simulink model "six_plus_six_AcmsteeringV09_main_1lf"  (R2014a)
settings: Solver=FixedStepDiscrete  StartTime=0.0  StopTime=10.0  FixedStep=0.0005  RelTol=1e-3
InitFcn:
  | Veh_Par_wxt
undefined symbols (not defined in the file or in its folder): acc_spdctl, ag_thr, B, bra_em, bra_pre_gz2, bra_pre_gz34, bra_pre_yd, brakepre_dem_data, brakeTrq_dem_data, bratrq_max, ecucoder_acal, eff_tran, ESP_switch, G, guzhang_lf, guzhang_lm, guzhang_lr, guzhang_rf, guzhang_rm, guzhang_rr, kd1, kd2, ki1, ki2, kp1, kp2, L, myFIS, premax, Radius, RC_switch, s_opt_yi, s_opt_zhuan, s_opt_zhuan_add, s_opt_zhuan_table, spd_map_mot, spd_spdctl, speed_thr_park, TCS_switch, tras_ratio, trq_map_mot, trqmax_yd, trqmax_zx, trqmaxneg, v_gain, v_table, v_thr_park, zhidong_bianmazhi, zhidong_down, zhidong_up, zhidong_youmen, zhuanxiang_bianmazhi, zhuanxiang_down, zhuanxiang_up, zhuanxiang_youmen
libraries: simulink x980, ec5744lib x59, fuzblock x2
(part 22 of 25)

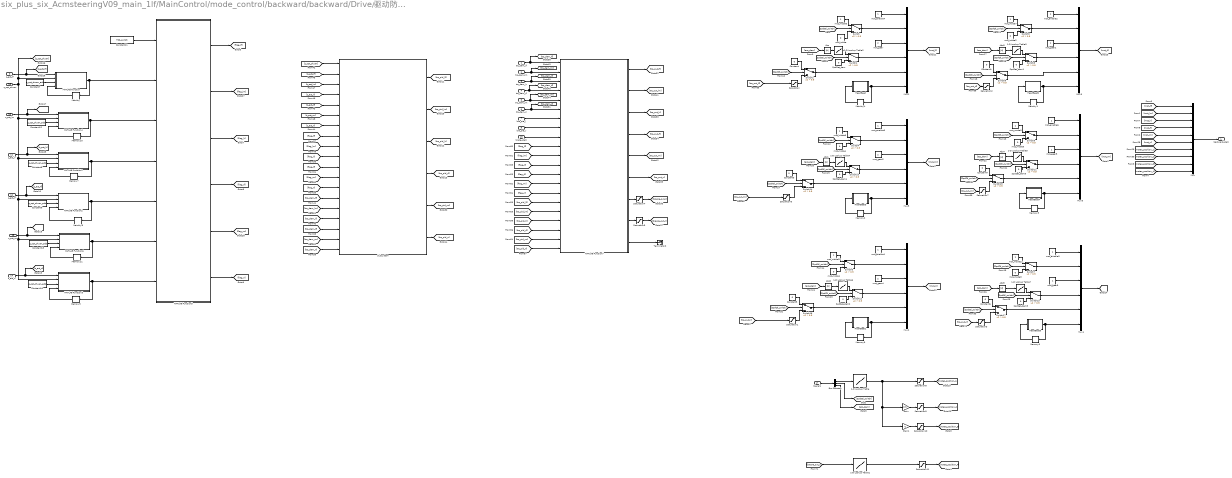
== system six_plus_six_AcmsteeringV09_main_1lf/MainControl/mode_control/backward/backward/Drive/驱动防滑控制TCS/直行TCS/直行 ==
  trq_dem_lf : Inport
  trq_dem_lm : Inport  Port=2
  trq_dem_lr : Inport  Port=3
  trq_dem_rf : Inport  Port=4
  trq_dem_rm : Inport  Port=5
  trq_dem_rr : Inport  Port=6
  bra_pre_l : Inport  Port=7
  bra_pre_r : Inport  Port=8
  s_act_lf : Inport  Port=9
  s_act_lm : Inport  Port=10
  s_act_lr : Inport  Port=11
  s_act_rf : Inport  Port=12
  s_act_rm : Inport  Port=13
  s_act_rr : Inport  Port=14
  brake_dem : Inport  Port=15
  s_opt_zhuan : Inport  Port=16
  Signals : Inport  Port=17
  1-D Lookup Table : Lookup_n-D  NumberOfTableDimensions=1  BreakpointsForDimension1=zhuanxiang_youmen  Table=zhuanxiang_bianmazhi  InternalRulePriority=Speed  RndMeth=Simplest  InputSameDT=on
  1-D Lookup Table1 : Lookup_n-D  NumberOfTableDimensions=1  BreakpointsForDimension1=zhidong_youmen  Table=zhidong_bianmazhi  InternalRulePriority=Speed  RndMeth=Simplest  InputSameDT=on
  1-D Lookup Table{2..7} (6 alike) : Lookup_n-D  NumberOfTableDimensions=1  BreakpointsForDimension1=acc_spdctl  Table=spd_spdctl  InternalRulePriority=Speed  RndMeth=Simplest  InputSameDT=on
  Abs{,1..5} (6 alike) : Abs
  Bus Selector : BusSelector  OutputSignals=RemoteControl_dem.steer_dem,RemoteControl_dem.SpdCtl_switch,RemoteControl_dem.acc_dem
  Constant{,1,3..6} (6 alike) : Constant  Value=0  OutDataTypeStr=single  SampleTime=-1
  Constant{7..10,12..13} (6 alike) : Constant  Value=s_opt_zhuan_add  OutDataTypeStr=single  SampleTime=-1
  Constant11 : Constant  Value=TCS_switch  OutDataTypeStr=single  SampleTime=-1
  Gain : Gain  Gain=0.5
  Gain1 : Gain  Gain=-1
  HeartBeat : MATLAB Function  TreatAsAtomicUnit=on
  HeartBeat1 : MATLAB Function  TreatAsAtomicUnit=on
  HeartBeat2 : MATLAB Function  TreatAsAtomicUnit=on
  HeartBeat3 : MATLAB Function  TreatAsAtomicUnit=on
  HeartBeat4 : MATLAB Function  TreatAsAtomicUnit=on
  HeartBeat5 : MATLAB Function  TreatAsAtomicUnit=on
  MATLAB Function : MATLAB Function  TreatAsAtomicUnit=on
  MATLAB Function1 : MATLAB Function  TreatAsAtomicUnit=on
  MATLAB Function2 : MATLAB Function  TreatAsAtomicUnit=on
  MATLAB Function3 : MATLAB Function  TreatAsAtomicUnit=on
  MATLAB Function4 : MATLAB Function  TreatAsAtomicUnit=on
  MATLAB Function5 : MATLAB Function  TreatAsAtomicUnit=on
  MATLAB Function6 : MATLAB Function  TreatAsAtomicUnit=on
  MATLAB Function7 : MATLAB Function  TreatAsAtomicUnit=on
  Memory{,1..11} (12 alike) : Memory  InheritSampleTime=on
  Mux : Mux  Inputs=10
  Mux{1..6} (6 alike) : Mux  Inputs=6
  Saturation{,1..3,6..7} (6 alike) : Saturate  UpperLimit=trqmax_zx  LowerLimit=trqmaxneg  OutDataTypeStr=single
  Saturation10 : Saturate  UpperLimit=zhuanxiang_up  LowerLimit=zhuanxiang_down
  Saturation11 : Saturate  UpperLimit=zhidong_up  LowerLimit=zhidong_down
  Saturation4 : Saturate  UpperLimit=premax  LowerLimit=0
  Saturation5 : Saturate  UpperLimit=premax  LowerLimit=0
  Saturation8 : Saturate  UpperLimit=zhuanxiang_up  LowerLimit=zhuanxiang_down
  Saturation9 : Saturate  UpperLimit=zhuanxiang_up  LowerLimit=zhuanxiang_down
  SpdSet_dem{,1..5} (6 alike) : Constant  Value=0  OutDataTypeStr=single  SampleTime=-1
  Subsystem : Subsystem
  Switch{,1..17} (18 alike) : Switch  Criteria=u2 > Threshold  Threshold=0.5
  Terminator2 : Terminator
  mot_enable{1..6} (6 alike) : Constant  OutDataTypeStr=single  SampleTime=-1
  mot_gear : Constant  Value=2  OutDataTypeStr=single  SampleTime=-1
  mot_gear1 : Constant  OutDataTypeStr=single  SampleTime=-1
  mot_gear2 : Constant  Value=2  OutDataTypeStr=single  SampleTime=-1
  mot_gear3 : Constant  OutDataTypeStr=single  SampleTime=-1
  mot_gear4 : Constant  Value=2  OutDataTypeStr=single  SampleTime=-1
  mot_gear5 : Constant  OutDataTypeStr=single  SampleTime=-1
  mot_mode{,1..5} (6 alike) : Constant  Value=0  OutDataTypeStr=single  SampleTime=-1
  mot_mode{6..11} (6 alike) : Constant  OutDataTypeStr=single  SampleTime=-1
  backward_dem : Outport
  wires:
  Mux/1 -> backward_dem/1
  Memory4/1 -> HeartBeat/1(life_pre)
  HeartBeat/1(life) -> Memory4/1, Mux1/6
  Mux1/1 -> [mot_lf]
  [trq_out_lf] -> Saturation/1
  mot_gear/1 -> Mux1/3
  mot_enable4/1 -> Mux1/1
  Switch1/1 -> Mux1/4
  Memory1/1 -> HeartBeat2/1(life_pre)
  HeartBeat2/1(life) -> Mux3/6, Memory1/1
  Mux3/1 -> [mot_rf]
  [trq_out_rf] -> Saturation2/1
  Switch3/1 -> Mux3/2
  mot_gear1/1 -> Mux3/3
  mot_enable2/1 -> Mux3/1
  Switch8/1 -> Mux3/4
  Memory2/1 -> HeartBeat3/1(life_pre)
  HeartBeat3/1(life) -> Mux5/6, Memory2/1
  Mux5/1 -> [mot_lm]
  [trq_out_lm] -> Saturation6/1
  Switch4/1 -> Mux5/2
  mot_gear2/1 -> Mux5/3
  mot_enable5/1 -> Mux5/1
  Switch10/1 -> Mux5/4
  Memory3/1 -> HeartBeat4/1(life_pre)
  HeartBeat4/1(life) -> Memory3/1, Mux6/6
  Mux6/1 -> [mot_rm]
  [trq_out_rm] -> Saturation7/1
  Switch5/1 -> Mux6/2
  mot_gear3/1 -> Mux6/3
  mot_enable6/1 -> Mux6/1
  Switch11/1 -> Mux6/4
  Memory5/1 -> HeartBeat1/1(life_pre)
  HeartBeat1/1(life) -> Mux2/6, Memory5/1
  Mux2/1 -> [mot_lr]
  [trq_out_lr] -> Saturation1/1
  Switch6/1 -> Mux2/2
  mot_gear4/1 -> Mux2/3
  mot_enable1/1 -> Mux2/1
  Switch12/1 -> Mux2/4
  Memory6/1 -> HeartBeat5/1(life_pre)
  HeartBeat5/1(life) -> Memory6/1, Mux4/6
  Mux4/1 -> [mot_rr]
  [trq_out_rr] -> Saturation3/1
  Switch7/1 -> Mux4/2
  mot_gear5/1 -> Mux4/3
  mot_enable3/1 -> Mux4/1
  Switch13/1 -> Mux4/4
  [mot_lf] -> Mux/1
  [mot_lm] -> Mux/2
  [mot_lr] -> Mux/3
  [mot_rf] -> Mux/4
  [mot_rm] -> Mux/5
  [mot_rr] -> Mux/6
  [motec_position_1] -> Mux/7
  [motec_position_2] -> Mux/8
  [motec_position_3] -> Mux/9
  1-D Lookup Table1/1 -> Saturation11/1
  1-D Lookup Table/1 -> Gain1/1, Gain/1, Saturation8/1
  Signals/1 -> Bus Selector/1
  Gain1/1 -> Saturation10/1
  Bus Selector/1 -> 1-D Lookup Table/1  "<steer_dem>"
  Gain/1 -> Saturation9/1
  Saturation8/1 -> [motec_position_1]
  Saturation9/1 -> [motec_position_2]
  Saturation10/1 -> [motec_position_3]
  Saturation11/1 -> [motec_position_4]
  [brapre_out_l] -> 1-D Lookup Table1/1
  [motec_position_4] -> Mux/10
  Bus Selector/2 -> [SpdCtl_switch]  "<SpdCtl_switch>"
  [SpdCtl_switch] -> Switch/2
  mot_mode6/1 -> Switch/1
  mot_mode/1 -> Switch/3
  Switch/1 -> Mux1/2
  [SpdCtl_switch] -> Switch1/2
  SpdSet_dem/1 -> Switch1/3
  Bus Selector/3 -> [acc_dem]  "<acc_dem>"
  [acc_dem] -> Abs/1
  1-D Lookup Table2/1 -> Switch1/1
  [SpdCtl_switch] -> Switch2/2
  Saturation/1 -> Switch2/3
  Constant/1 -> Switch2/1
  Switch2/1 -> Mux1/5
  [SpdCtl_switch] -> Switch3/2
  mot_mode7/1 -> Switch3/1
  mot_mode2/1 -> Switch3/3
  [SpdCtl_switch] -> Switch4/2
  mot_mode8/1 -> Switch4/1
  mot_mode4/1 -> Switch4/3
  [SpdCtl_switch] -> Switch5/2
  mot_mode9/1 -> Switch5/1
  mot_mode5/1 -> Switch5/3
  [SpdCtl_switch] -> Switch6/2
  mot_mode10/1 -> Switch6/1
  mot_mode1/1 -> Switch6/3
  [SpdCtl_switch] -> Switch7/2
  mot_mode11/1 -> Switch7/1
  mot_mode3/1 -> Switch7/3
  [SpdCtl_switch] -> Switch8/2
  [acc_dem] -> Abs3/1
  1-D Lookup Table3/1 -> Switch8/1
  SpdSet_dem1/1 -> Switch8/3
  [SpdCtl_switch] -> Switch9/2
  Constant1/1 -> Switch9/1
  Saturation2/1 -> Switch9/3
  Switch9/1 -> Mux3/5
  [SpdCtl_switch] -> Switch10/2
  [acc_dem] -> Abs1/1
  1-D Lookup Table4/1 -> Switch10/1
  SpdSet_dem4/1 -> Switch10/3
  [SpdCtl_switch] -> Switch11/2
  [acc_dem] -> Abs4/1
  1-D Lookup Table5/1 -> Switch11/1
  SpdSet_dem5/1 -> Switch11/3
  [SpdCtl_switch] -> Switch12/2
  [acc_dem] -> Abs2/1
  1-D Lookup Table6/1 -> Switch12/1
  SpdSet_dem2/1 -> Switch12/3
  [SpdCtl_switch] -> Switch13/2
  [acc_dem] -> Abs5/1
  1-D Lookup Table7/1 -> Switch13/1
  SpdSet_dem3/1 -> Switch13/3
  [SpdCtl_switch] -> Switch14/2
  Constant3/1 -> Switch14/1
  Saturation6/1 -> Switch14/3
  Switch14/1 -> Mux5/5
  [SpdCtl_switch] -> Switch15/2
  Constant4/1 -> Switch15/1
  Saturation7/1 -> Switch15/3
  Switch15/1 -> Mux6/5
  [SpdCtl_switch] -> Switch16/2
  Constant5/1 -> Switch16/1
  Saturation1/1 -> Switch16/3
  Switch16/1 -> Mux2/5
  [SpdCtl_switch] -> Switch17/2
  Constant6/1 -> Switch17/1
  Saturation3/1 -> Switch17/3
  Switch17/1 -> Mux4/5
  Constant10/1 -> MATLAB Function3/3(s_opt_zhuan_add)
  Memory9/1 -> MATLAB Function3/4(flag_rr_pre)
  MATLAB Function3/1(flag_rr) -> Memory9/1, MATLAB Function5/7(flag_rr)
  s_act_rr/1 -> [s_act_rr], MATLAB Function3/1(s_act_rr)
  Constant9/1 -> MATLAB Function2/3(s_opt_zhuan_add)
  Memory8/1 -> MATLAB Function2/4(flag_rf_pre)
  MATLAB Function2/1(flag_rf) -> Memory8/1, MATLAB Function5/5(flag_rf)
  s_act_rf/1 -> MATLAB Function2/1(s_act_rf), [s_act_rf]
  Constant8/1 -> MATLAB Function1/3(s_opt_zhuan_add)
  Memory7/1 -> MATLAB Function1/4(flag_lr_pre)
  MATLAB Function1/1(flag_lr) -> Memory7/1, MATLAB Function5/4(flag_lr)
  s_act_lr/1 -> [s_act_lr], MATLAB Function1/1(s_act_lr)
  Constant7/1 -> MATLAB Function/3(s_opt_zhuan_add)
  Memory/1 -> MATLAB Function/4(flag_lf_pre)
  MATLAB Function/1(flag_lf) -> Memory/1, MATLAB Function5/2(flag_lf)
  s_act_lf/1 -> [s_act_lf], MATLAB Function/1(s_act_lf)
  [trq_dem_lf] -> Subsystem/14(trq_dem_lf)
  [flag_lf] -> Subsystem/8(flag_lf)
  [trq_dem_rf] -> Subsystem/17(trq_dem_rf)
  [trq_dem_lr] -> Subsystem/16(trq_dem_lr)
  [flag_lr] -> Subsystem/10(flag_lr)
  [flag_rf] -> Subsystem/11(flag_rf)
  [trq_dem_rr] -> Subsystem/19(trq_dem_rr)
  [flag_rr] -> Subsystem/13(flag_rr)
  [s_opt_zhuan] -> Subsystem/1(s_opt_zhuan)
  [s_act_rr] -> Subsystem/7(s_act_rr)
  [s_act_rf] -> Subsystem/5(s_act_rf)
  [s_act_lr] -> Subsystem/4(s_act_lr)
  [s_act_lf] -> Subsystem/2(s_act_lf)
  Subsystem/3(trq_pid_lr) -> [trq_pid_lr]
  Subsystem/1(trq_pid_lf) -> [trq_pid_lf]
  Subsystem/6(trq_pid_rr) -> [trq_pid_rr]
  Subsystem/4(trq_pid_rf) -> [trq_pid_rf]
  MATLAB Function5/1(flag_lf1) -> [flag_lf]
  MATLAB Function5/3(flag_lr1) -> [flag_lr]
  MATLAB Function5/4(flag_rf1) -> [flag_rf]
  MATLAB Function5/6(flag_rr1) -> [flag_rr]
  Constant12/1 -> MATLAB Function4/3(s_opt_zhuan_add)
  Memory10/1 -> MATLAB Function4/4(flag_lm_pre)
  MATLAB Function4/1(flag_lm) -> MATLAB Function5/3(flag_lm), Memory10/1
  s_act_lm/1 -> MATLAB Function4/1(s_act_lm), [s_act_lm]
  Constant13/1 -> MATLAB Function6/3(s_opt_zhuan_add)
  Memory11/1 -> MATLAB Function6/4(flag_rm_pre)
  MATLAB Function6/1(flag_rm) -> Memory11/1, MATLAB Function5/6(flag_rm)
  s_act_rm/1 -> [s_act_rm], MATLAB Function6/1(s_act_rm)
  s_opt_zhuan/1 -> MATLAB Function/2(s_opt_zhuan), [s_opt_zhuan], MATLAB Function4/2(s_opt_zhuan), MATLAB Function1/2(s_opt_zhuan), MATLAB Function2/2(s_opt_zhuan), MATLAB Function6/2(s_opt_zhuan), MATLAB Function3/2(s_opt_zhuan)
  MATLAB Function5/2(flag_lm1) -> [flag_lm]
  MATLAB Function5/5(flag_rm1) -> [flag_rm]
  Constant11/1 -> MATLAB Function5/1(TCS_switch)
  [s_act_lm] -> Subsystem/3(s_act_lm)
  [s_act_rm] -> Subsystem/6(s_act_rm)
  [flag_lm] -> Subsystem/9(flag_lm)
  [flag_rm] -> Subsystem/12(flag_rm)
  [trq_dem_lm] -> Subsystem/15(trq_dem_lm)
  [trq_dem_rm] -> Subsystem/18(trq_dem_rm)
  Subsystem/2(trq_pid_lm) -> [trq_pid_lm]
  Subsystem/5(trq_pid_rm) -> [trq_pid_rm]
  [flag_rr] -> MATLAB Function7/15(flag_rr)
  [flag_rf] -> MATLAB Function7/13(flag_rf)
  [flag_lr] -> MATLAB Function7/12(flag_lr)
  [flag_lf] -> MATLAB Function7/10(flag_lf)
  [trq_pid_lf] -> MATLAB Function7/16(trq_pid_lf)
  [trq_pid_lr] -> MATLAB Function7/18(trq_pid_lr)
  [trq_pid_rf] -> MATLAB Function7/19(trq_pid_rf)
  [trq_pid_rr] -> MATLAB Function7/21(trq_pid_rr)
  trq_dem_lf/1 -> MATLAB Function7/1(trq_dem_lf), [trq_dem_lf]
  trq_dem_lr/1 -> [trq_dem_lr], MATLAB Function7/3(trq_dem_lr)
  trq_dem_rf/1 -> MATLAB Function7/4(trq_dem_rf), [trq_dem_rf]
  trq_dem_rr/1 -> [trq_dem_rr], MATLAB Function7/6(trq_dem_rr)
  bra_pre_l/1 -> MATLAB Function7/7(bra_pre_l)
  bra_pre_r/1 -> MATLAB Function7/8(bra_pre_r)
  MATLAB Function7/1(trq_out_lf) -> [trq_out_lf]
  MATLAB Function7/3(trq_out_lr) -> [trq_out_lr]
  MATLAB Function7/4(trq_out_rf) -> [trq_out_rf]
  MATLAB Function7/6(trq_out_rr) -> [trq_out_rr]
  MATLAB Function7/7(brapre_out_l) -> Saturation4/1
  MATLAB Function7/8(brapre_out_r) -> Saturation5/1
  brake_dem/1 -> MATLAB Function7/9(brake_dem)
  MATLAB Function7/9(mode) -> Terminator2/1
  Saturation4/1 -> [brapre_out_l]
  Saturation5/1 -> [brapre_out_r]
  MATLAB Function7/2(trq_out_lm) -> [trq_out_lm]
  MATLAB Function7/5(trq_out_rm) -> [trq_out_rm]
  trq_dem_lm/1 -> [trq_dem_lm], MATLAB Function7/2(trq_dem_lm)
  trq_dem_rm/1 -> [trq_dem_rm], MATLAB Function7/5(trq_dem_rm)
  [flag_lm] -> MATLAB Function7/11(flag_lm)
  [flag_rm] -> MATLAB Function7/14(flag_rm)
  [trq_pid_lm] -> MATLAB Function7/17(trq_pid_lm)
  [trq_pid_rm] -> MATLAB Function7/20(trq_pid_rm)
  Abs/1 -> 1-D Lookup Table2/1
  Abs1/1 -> 1-D Lookup Table4/1
  Abs2/1 -> 1-D Lookup Table6/1
  Abs3/1 -> 1-D Lookup Table3/1
  Abs4/1 -> 1-D Lookup Table5/1
  Abs5/1 -> 1-D Lookup Table7/1

== system six_plus_six_AcmsteeringV09_main_1lf/MainControl/mode_control/forward/forward/Drive/驱动防滑控制TCS/直行TCS/Subsystem ==
  speed_act_lf : Inport
  v_act : Inport  Port=2
  Add : Sum
  Constant : Constant  Value=eps  OutDataTypeStr=single  SampleTime=-1
  Divide : Product  Inputs=*/
  Gain : Gain  Gain=pi/30
  Gain1 : Gain  Gain=Radius
  Gain2 : Gain  Gain=1/3.6
  Gain3 : Gain  Gain=1/tras_ratio
  Subtract : Sum  Inputs=+-
  s_act_lf : Outport
  wires:
  Divide/1 -> s_act_lf/1
  Add/1 -> Divide/2
  Constant/1 -> Add/2
  Subtract/1 -> Divide/1
  Gain1/1 -> Subtract/1, Add/1
  v_act/1 -> Gain2/1
  Gain/1 -> Gain1/1
  speed_act_lf/1 -> Gain3/1
  Gain3/1 -> Gain/1
  Gain2/1 -> Subtract/2

== system six_plus_six_AcmsteeringV09_main_1lf/MainControl/mode_control/forward/forward/Drive/驱动防滑控制TCS/直行TCS/Subsystem1 ==
  speed_act_lm : Inport
  v_act : Inport  Port=2
  Add : Sum
  Constant : Constant  Value=eps  OutDataTypeStr=single  SampleTime=-1
  Divide : Product  Inputs=*/
  Gain : Gain  Gain=pi/30
  Gain1 : Gain  Gain=Radius
  Gain2 : Gain  Gain=1/3.6
  Gain3 : Gain  Gain=1/tras_ratio
  Subtract : Sum  Inputs=+-
  s_act_lm : Outport
  wires:
  Gain2/1 -> Subtract/2
  Gain3/1 -> Gain/1
  speed_act_lm/1 -> Gain3/1
  Gain/1 -> Gain1/1
  v_act/1 -> Gain2/1
  Gain1/1 -> Add/1, Subtract/1
  Subtract/1 -> Divide/1
  Constant/1 -> Add/2
  Add/1 -> Divide/2
  Divide/1 -> s_act_lm/1

== system six_plus_six_AcmsteeringV09_main_1lf/MainControl/mode_control/forward/forward/Drive/驱动防滑控制TCS/直行TCS/Subsystem2 ==
  speed_act_lr : Inport
  v_act : Inport  Port=2
  Add : Sum
  Constant : Constant  Value=eps  OutDataTypeStr=single  SampleTime=-1
  Divide : Product  Inputs=*/
  Gain : Gain  Gain=pi/30
  Gain1 : Gain  Gain=Radius
  Gain2 : Gain  Gain=1/3.6
  Gain3 : Gain  Gain=1/tras_ratio
  Subtract : Sum  Inputs=+-
  s_act_lr : Outport
  wires:
  Gain2/1 -> Subtract/2
  Gain3/1 -> Gain/1
  speed_act_lr/1 -> Gain3/1
  Gain/1 -> Gain1/1
  v_act/1 -> Gain2/1
  Gain1/1 -> Add/1, Subtract/1
  Subtract/1 -> Divide/1
  Constant/1 -> Add/2
  Add/1 -> Divide/2
  Divide/1 -> s_act_lr/1

== system six_plus_six_AcmsteeringV09_main_1lf/MainControl/mode_control/forward/forward/Drive/驱动防滑控制TCS/直行TCS/Subsystem3 ==
  speed_act_rf : Inport
  v_act : Inport  Port=2
  Add : Sum
  Constant : Constant  Value=eps  OutDataTypeStr=single  SampleTime=-1
  Divide : Product  Inputs=*/
  Gain : Gain  Gain=pi/30
  Gain1 : Gain  Gain=Radius
  Gain2 : Gain  Gain=1/3.6
  Gain3 : Gain  Gain=1/tras_ratio
  Subtract : Sum  Inputs=+-
  s_act_rf : Outport
  wires:
  Divide/1 -> s_act_rf/1
  Add/1 -> Divide/2
  Constant/1 -> Add/2
  Subtract/1 -> Divide/1
  Gain1/1 -> Subtract/1, Add/1
  v_act/1 -> Gain2/1
  Gain/1 -> Gain1/1
  speed_act_rf/1 -> Gain3/1
  Gain3/1 -> Gain/1
  Gain2/1 -> Subtract/2

== system six_plus_six_AcmsteeringV09_main_1lf/MainControl/mode_control/forward/forward/Drive/驱动防滑控制TCS/直行TCS/Subsystem4 ==
  speed_act_rm : Inport
  v_act : Inport  Port=2
  Add : Sum
  Constant : Constant  Value=eps  OutDataTypeStr=single  SampleTime=-1
  Divide : Product  Inputs=*/
  Gain : Gain  Gain=pi/30
  Gain1 : Gain  Gain=Radius
  Gain2 : Gain  Gain=1/3.6
  Gain3 : Gain  Gain=1/tras_ratio
  Subtract : Sum  Inputs=+-
  s_act_rm : Outport
  wires:
  Gain2/1 -> Subtract/2
  Gain3/1 -> Gain/1
  speed_act_rm/1 -> Gain3/1
  Gain/1 -> Gain1/1
  v_act/1 -> Gain2/1
  Gain1/1 -> Add/1, Subtract/1
  Subtract/1 -> Divide/1
  Constant/1 -> Add/2
  Add/1 -> Divide/2
  Divide/1 -> s_act_rm/1

== system six_plus_six_AcmsteeringV09_main_1lf/MainControl/mode_control/forward/forward/Drive/驱动防滑控制TCS/直行TCS/Subsystem5 ==
  speed_act_rr : Inport
  v_act : Inport  Port=2
  Add : Sum
  Constant : Constant  Value=eps  OutDataTypeStr=single  SampleTime=-1
  Divide : Product  Inputs=*/
  Gain : Gain  Gain=pi/30
  Gain1 : Gain  Gain=Radius
  Gain2 : Gain  Gain=1/3.6
  Gain3 : Gain  Gain=1/tras_ratio
  Subtract : Sum  Inputs=+-
  s_act_rr : Outport
  wires:
  Divide/1 -> s_act_rr/1
  Add/1 -> Divide/2
  Constant/1 -> Add/2
  Subtract/1 -> Divide/1
  Gain1/1 -> Subtract/1, Add/1
  v_act/1 -> Gain2/1
  Gain/1 -> Gain1/1
  speed_act_rr/1 -> Gain3/1
  Gain3/1 -> Gain/1
  Gain2/1 -> Subtract/2

== system six_plus_six_AcmsteeringV09_main_1lf/MainControl/mode_control/forward/forward/Drive/驱动防滑控制TCS/直行TCS/Subsystem6 ==
  speed_act_lf : Inport
  speed_act_lm : Inport  Port=2
  speed_act_lr : Inport  Port=3
  Gain : Gain  Gain=1/tras_ratio
  Gain1 : Gain  Gain=pi/30
  Gain2 : Gain  Gain=Radius
  Gain3 : Gain  Gain=3.6
  Gain4 : Gain  Gain=v_gain
  MinMax : MinMax  Inputs=3
  v_act_l : Outport
  wires:
  speed_act_lm/1 -> MinMax/2
  speed_act_lr/1 -> MinMax/3
  speed_act_lf/1 -> MinMax/1
  MinMax/1 -> Gain/1
  Gain/1 -> Gain1/1
  Gain1/1 -> Gain2/1
  Gain2/1 -> Gain3/1
  Gain3/1 -> Gain4/1
  Gain4/1 -> v_act_l/1

== system six_plus_six_AcmsteeringV09_main_1lf/MainControl/mode_control/forward/forward/Drive/驱动防滑控制TCS/直行TCS/Subsystem7 ==
  speed_act_rf : Inport
  speed_act_rm : Inport  Port=2
  speed_act_rr : Inport  Port=3
  Gain : Gain  Gain=1/tras_ratio
  Gain1 : Gain  Gain=pi/30
  Gain2 : Gain  Gain=Radius
  Gain3 : Gain  Gain=3.6
  Gain4 : Gain  Gain=v_gain
  MinMax : MinMax  Inputs=3
  v_act_r : Outport
  wires:
  Gain4/1 -> v_act_r/1
  Gain3/1 -> Gain4/1
  Gain2/1 -> Gain3/1
  Gain1/1 -> Gain2/1
  Gain/1 -> Gain1/1
  MinMax/1 -> Gain/1
  speed_act_rf/1 -> MinMax/1
  speed_act_rr/1 -> MinMax/3
  speed_act_rm/1 -> MinMax/2

== matlab function six_plus_six_AcmsteeringV09_main_1lf/MainControl/mode_control/neutral/neutral/HeartBeat ==
  data: life_pre input; life output
function life = fcn(life_pre)
%#codegen
life=single(life_pre+1);
if life>255
    life=single(0);
end
end

== matlab function six_plus_six_AcmsteeringV09_main_1lf/Data_input/3/Enabled Subsystem/MATLAB Function3 ==
  data: speed input; speed_out output
function speed_out = motec_speed(speed)
    if speed>32768
        speed_out=speed-65535;
    else speed_out=speed;
    end
end

== matlab function six_plus_six_AcmsteeringV09_main_1lf/MainControl/mode_control/neutral/neutral/HeartBeat3 ==
  data: life_pre input; life output
function life = fcn(life_pre)
%#codegen
life=single(life_pre+1);
if life>255
    life=single(0);
end
end

== matlab function six_plus_six_AcmsteeringV09_main_1lf/MainControl/mode_control/backward/backward/Brake/HeartBeat1 ==
  data: life_pre input; life output
function life = fcn(life_pre)
%#codegen
life=single(life_pre+1);
if life>255
    life=single(0);
end
end

== matlab function six_plus_six_AcmsteeringV09_main_1lf/MainControl/mode_control/backward/backward/Brake/HeartBeat3 ==
  data: life_pre input; life output
function life = fcn(life_pre)
%#codegen
life=single(life_pre+1);
if life>255
    life=single(0);
end
end

== matlab function six_plus_six_AcmsteeringV09_main_1lf/MainControl/mode_control/backward/backward/Brake/HeartBeat5 ==
  data: life_pre input; life output
function life = fcn(life_pre)
%#codegen
life=single(life_pre+1);
if life>255
    life=single(0);
end
end
